simulink model "w2Problem2"  (R2020b)
settings: Solver=ode23  StartTime=0.0  StopTime=10.0  RelTol=1e-3
PostLoadFcn:
  | open_Building_a_Clutch_Lock_Up_Model
undefined symbols (not defined in the file): be, bv, Ie, Iv, muk, mus, R
CloseFcn:
  | close open_Building_a_Clutch_Lock_Up_Model
settings Model: DataDictionary=w2p2_data.sldd  Creator=k.Raviteja  LastModifiedBy=k.Raviteja
settings SolverCC: ZeroCrossAlgorithm=Adaptive
settings DebuggingCC: MaskedZcDiagnostic=none  IgnoredZcDiagnostic=none

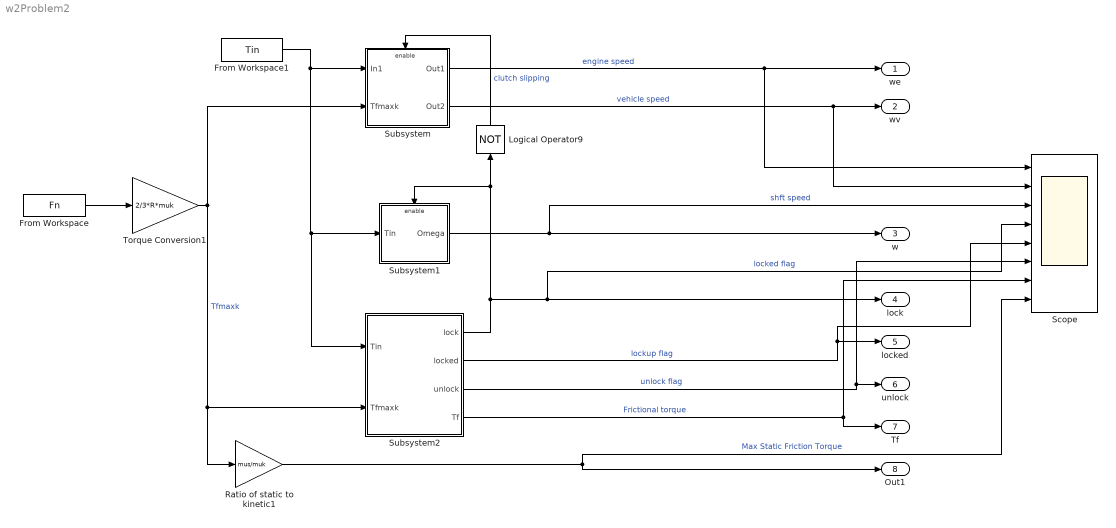
== system w2Problem2 ==
  From Workspace : FromWorkspace  VariableName=Fn  ZeroCross=off
  From Workspace1 : FromWorkspace  VariableName=Tin  ZeroCross=off
  Logical Operator9 : Logic  Operator=NOT  Inputs=1  IconShape=distinctive  OutDataTypeStr=boolean
  Ratio of static to kinetic1 : Gain  Gain=mus/muk  SaturateOnIntegerOverflow=on  OutDataTypeStr=Inherit: Same as input  ParamDataTypeStr=Inherit: Same as input
  Scope : Scope  NumInputPorts=8
  Subsystem : Subsystem
  Subsystem1 : Subsystem
  Subsystem2 : Subsystem
  Torque Conversion1 : Gain  Gain=2/3*R*muk  SaturateOnIntegerOverflow=on  OutDataTypeStr=Inherit: Same as input  ParamDataTypeStr=Inherit: Same as input
  we : Outport  InitialOutput=0  VectorParamsAs1DForOutWhenUnconnected=off
  wv : Outport  Port=2  InitialOutput=0  VectorParamsAs1DForOutWhenUnconnected=off
  w : Outport  Port=3
  lock : Outport  Port=4
  locked : Outport  Port=5
  unlock : Outport  Port=6
  Tf : Outport  Port=7
  Out1 : Outport  Port=8
  wires:
  From Workspace/1 -> Torque Conversion1/1
  Torque Conversion1/1 -> Ratio of static to kinetic1/1, Subsystem2/2(Tfmaxk), Subsystem/2(Tfmaxk)  "Tfmaxk"
  Ratio of static to kinetic1/1 -> Out1/1, Scope/8  "Max Static Friction Torque"
  Subsystem/1(Out1) -> Scope/1, we/1  "engine speed"
  Subsystem/2(Out2) -> Scope/2, wv/1  "vehicle speed"
  Logical Operator9/1 -> Subsystem/Enable  "clutch slipping"
  Subsystem1/1(Omega) -> Scope/3, w/1  "shft speed"
  Subsystem2/1(lock) -> Scope/4, lock/1, Subsystem1/Enable, Logical Operator9/1  "locked flag"
  From Workspace1/1 -> Subsystem2/1(Tin), Subsystem1/1(Tin), Subsystem/1(In1)
  Subsystem2/2(locked) -> Scope/5, locked/1  "lockup flag"
  Subsystem2/3(unlock) -> Scope/6, unlock/1  "unlock flag"
  Subsystem2/4(Tf) -> Tf/1, Scope/7  "Frictional torque"

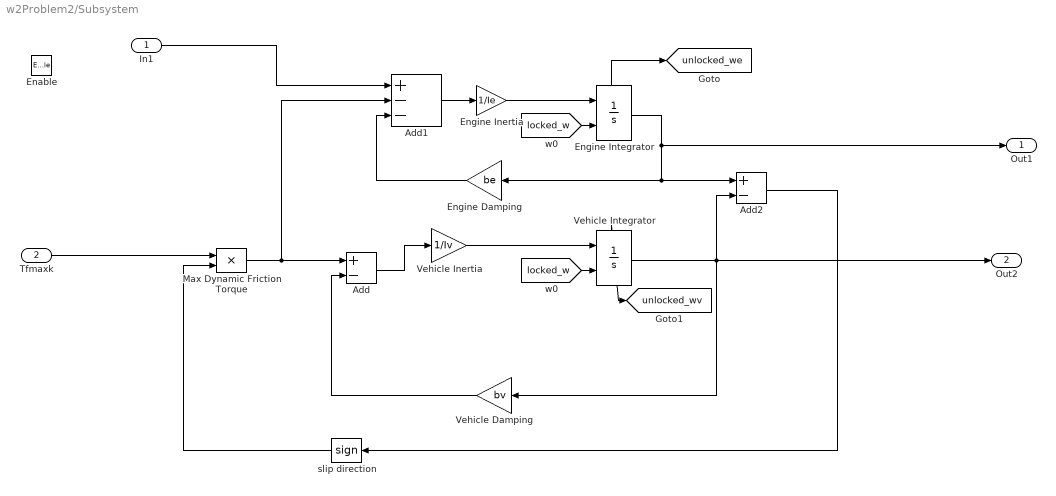
== system w2Problem2/Subsystem ==
  In1 : Inport
  Tfmaxk : Inport  Port=2
  Enable : EnablePort  StatesWhenEnabling=reset
  Add : Sum  Inputs=+-
  Add1 : Sum  Inputs=+--
  Add2 : Sum  Inputs=+-
  Engine Damping : Gain  Gain=be  SaturateOnIntegerOverflow=on  OutDataTypeStr=Inherit: Same as input  ParamDataTypeStr=Inherit: Same as input
  Engine Inertia : Gain  Gain=1/Ie  SaturateOnIntegerOverflow=on  OutDataTypeStr=Inherit: Same as input  ParamDataTypeStr=Inherit: Same as input
  Engine Integrator : Integrator  InitialConditionSource=external  ShowStatePort=on
  Max Dynamic Friction Torque : Product  InputSameDT=on  RndMeth=Zero  SaturateOnIntegerOverflow=on  OutDataTypeStr=Inherit: Same as first input
  Vehicle Damping : Gain  Gain=bv  SaturateOnIntegerOverflow=on  OutDataTypeStr=Inherit: Same as input  ParamDataTypeStr=Inherit: Same as input
  Vehicle Inertia : Gain  Gain=1/Iv  SaturateOnIntegerOverflow=on  OutDataTypeStr=Inherit: Same as input  ParamDataTypeStr=Inherit: Same as input
  Vehicle Integrator : Integrator  InitialConditionSource=external  ShowStatePort=on
  slip direction : Signum
  Out1 : Outport
  Out2 : Outport  Port=2
  tag scope: unlocked_we=global, unlocked_wv=global
  wires:
  [locked_w] -> Vehicle Integrator/2
  Engine Integrator/1 -> Out1/1, Engine Damping/1, Add2/1
  Vehicle Integrator/State -> [unlocked_wv]
  Engine Damping/1 -> Add1/3
  Add2/1 -> slip direction/1
  Max Dynamic Friction Torque/1 -> Add1/2, Add/1
  Engine Inertia/1 -> Engine Integrator/1
  [locked_w] -> Engine Integrator/2
  Vehicle Inertia/1 -> Vehicle Integrator/1
  Engine Integrator/State -> [unlocked_we]
  slip direction/1 -> Max Dynamic Friction Torque/2
  Vehicle Integrator/1 -> Out2/1, Add2/2, Vehicle Damping/1
  Add1/1 -> Engine Inertia/1
  Vehicle Damping/1 -> Add/2
  Add/1 -> Vehicle Inertia/1
  In1/1 -> Add1/1
  Tfmaxk/1 -> Max Dynamic Friction Torque/1

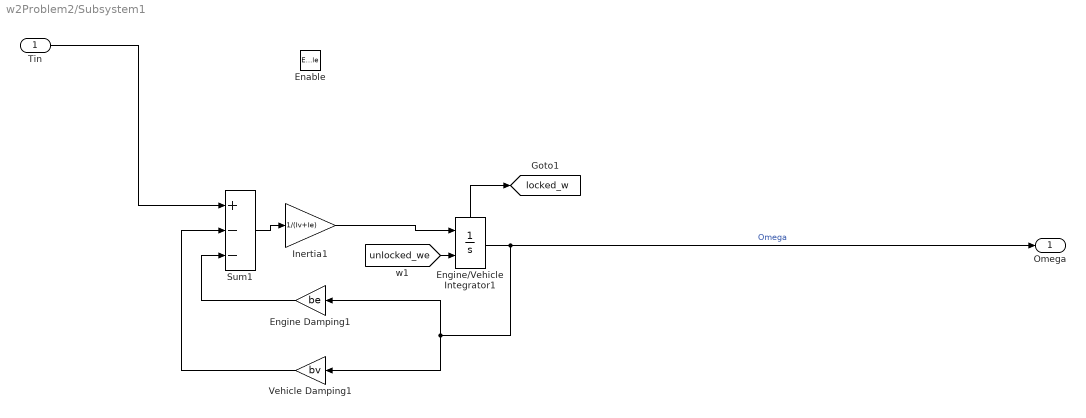
== system w2Problem2/Subsystem1 ==
  Tin : Inport
  Enable : EnablePort  StatesWhenEnabling=reset
  Engine Damping1 : Gain  Gain=be  SaturateOnIntegerOverflow=on  OutDataTypeStr=Inherit: Same as input  ParamDataTypeStr=Inherit: Same as input
  Engine/Vehicle Integrator1 : Integrator  InitialConditionSource=external  ShowStatePort=on
  Inertia1 : Gain  Gain=1/(Iv+Ie)  SaturateOnIntegerOverflow=on  OutDataTypeStr=Inherit: Same as input  ParamDataTypeStr=Inherit: Same as input
  Sum1 : Sum  Inputs=+--  InputSameDT=on  SaturateOnIntegerOverflow=on  OutDataTypeStr=Inherit: Same as first input
  Vehicle Damping1 : Gain  Gain=bv  SaturateOnIntegerOverflow=on  OutDataTypeStr=Inherit: Same as input  ParamDataTypeStr=Inherit: Same as input
  Omega : Outport
  tag scope: locked_w=global
  wires:
  Engine/Vehicle Integrator1/1 -> Omega/1, Engine Damping1/1, Vehicle Damping1/1  "Omega"
  [unlocked_we] -> Engine/Vehicle Integrator1/2
  Sum1/1 -> Inertia1/1
  Engine/Vehicle Integrator1/State -> [locked_w]
  Vehicle Damping1/1 -> Sum1/2
  Engine Damping1/1 -> Sum1/3
  Inertia1/1 -> Engine/Vehicle Integrator1/1
  Tin/1 -> Sum1/1

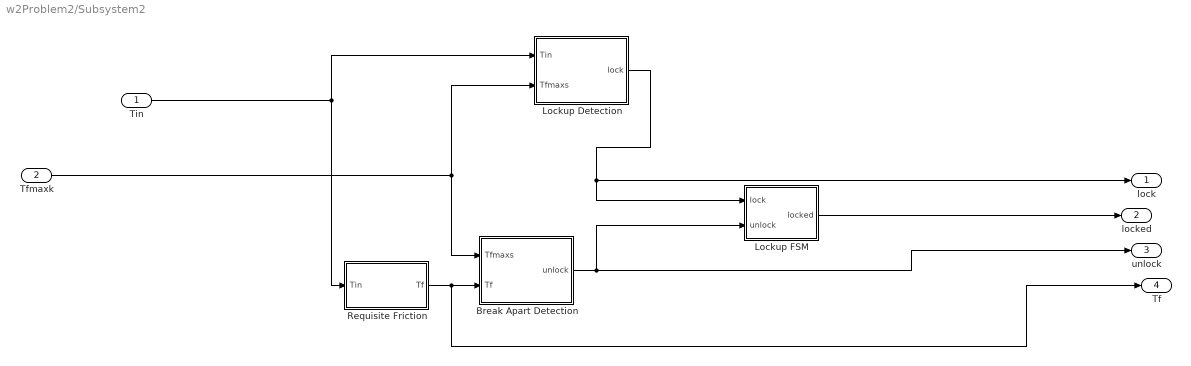
== system w2Problem2/Subsystem2 ==
  Tin : Inport
  Tfmaxk : Inport  Port=2
  Break Apart Detection : Subsystem
  Lockup Detection : Subsystem
  Lockup FSM : Subsystem
  Requisite Friction : Subsystem
  lock : Outport
  locked : Outport  Port=2
  unlock : Outport  Port=3
  Tf : Outport  Port=4
  wires:
  Break Apart Detection/1(unlock) -> unlock/1, Lockup FSM/2(unlock)
  Lockup Detection/1(lock) -> lock/1, Lockup FSM/1(lock)
  Tfmaxk/1 -> Break Apart Detection/1(Tfmaxs), Lockup Detection/2(Tfmaxs)
  Tin/1 -> Requisite Friction/1(Tin), Lockup Detection/1(Tin)
  Requisite Friction/1(Tf) -> Tf/1, Break Apart Detection/2(Tf)
  Lockup FSM/1(locked) -> locked/1

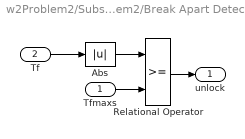
== system w2Problem2/Subsystem2/Break Apart Detection ==
  Tfmaxs : Inport
  Tf : Inport  Port=2
  Abs : Abs  SaturateOnIntegerOverflow=on
  Relational Operator : RelationalOperator  OutDataTypeStr=boolean  RndMeth=Nearest  InputSameDT=on
  unlock : Outport  InitialOutput=0  VectorParamsAs1DForOutWhenUnconnected=off
  wires:
  Tf/1 -> Abs/1
  Relational Operator/1 -> unlock/1
  Abs/1 -> Relational Operator/1
  Tfmaxs/1 -> Relational Operator/2

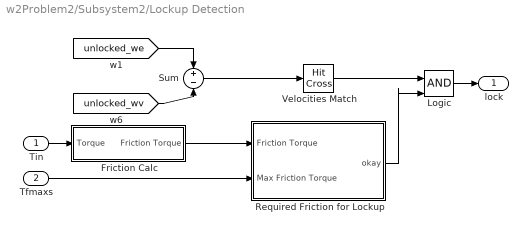
== system w2Problem2/Subsystem2/Lockup Detection ==
  Tin : Inport
  Tfmaxs : Inport  Port=2
  Friction Calc : Subsystem
  Logic : Logic  IconShape=distinctive  OutDataTypeStr=boolean
  Required Friction for Lockup : Subsystem
  Sum : Sum  Inputs=+-  InputSameDT=on  SaturateOnIntegerOverflow=on  OutDataTypeStr=Inherit: Same as first input
  Velocities Match : HitCross
  lock : Outport  InitialOutput=0  VectorParamsAs1DForOutWhenUnconnected=off
  wires:
  Friction Calc/1(Friction Torque) -> Required Friction for Lockup/1(Friction Torque)
  Tfmaxs/1 -> Required Friction for Lockup/2(Max Friction Torque)
  Velocities Match/1 -> Logic/1
  Logic/1 -> lock/1
  Required Friction for Lockup/1(okay) -> Logic/2
  [unlocked_we] -> Sum/1
  [unlocked_wv] -> Sum/2
  Sum/1 -> Velocities Match/1
  Tin/1 -> Friction Calc/1(Torque)

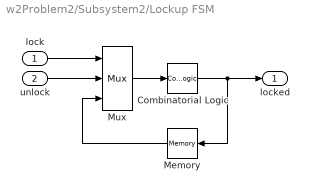
== system w2Problem2/Subsystem2/Lockup FSM ==
  lock : Inport
  unlock : Inport  Port=2
  Combinatorial Logic : CombinatorialLogic  TruthTable=[0;1;0;0;1;1;1;0]
  Memory : Memory
  Mux : Mux  Inputs=3
  locked : Outport  InitialOutput=0  VectorParamsAs1DForOutWhenUnconnected=off
  wires:
  Memory/1 -> Mux/3
  Combinatorial Logic/1 -> locked/1, Memory/1
  unlock/1 -> Mux/2
  lock/1 -> Mux/1
  Mux/1 -> Combinatorial Logic/1

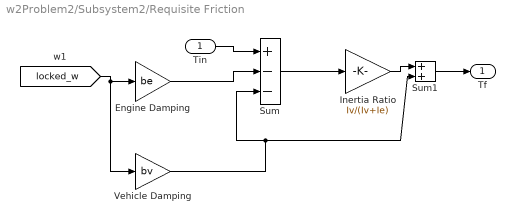
== system w2Problem2/Subsystem2/Requisite Friction ==
  Tin : Inport
  Engine Damping : Gain  Gain=be  SaturateOnIntegerOverflow=on  OutDataTypeStr=Inherit: Same as input  ParamDataTypeStr=Inherit: Same as input
  Inertia Ratio : Gain  Gain=Iv/(Iv+Ie)  SaturateOnIntegerOverflow=on  OutDataTypeStr=Inherit: Same as input  ParamDataTypeStr=Inherit: Same as input
  Sum : Sum  Inputs=+--  InputSameDT=on  SaturateOnIntegerOverflow=on  OutDataTypeStr=Inherit: Same as first input
  Sum1 : Sum  InputSameDT=on  SaturateOnIntegerOverflow=on  OutDataTypeStr=Inherit: Same as first input
  Vehicle Damping : Gain  Gain=bv  SaturateOnIntegerOverflow=on  OutDataTypeStr=Inherit: Same as input  ParamDataTypeStr=Inherit: Same as input
  Tf : Outport  InitialOutput=0  VectorParamsAs1DForOutWhenUnconnected=off
  wires:
  [locked_w] -> Vehicle Damping/1, Engine Damping/1
  Engine Damping/1 -> Sum/2
  Vehicle Damping/1 -> Sum/3, Sum1/2
  Sum/1 -> Inertia Ratio/1
  Tin/1 -> Sum/1
  Inertia Ratio/1 -> Sum1/1
  Sum1/1 -> Tf/1

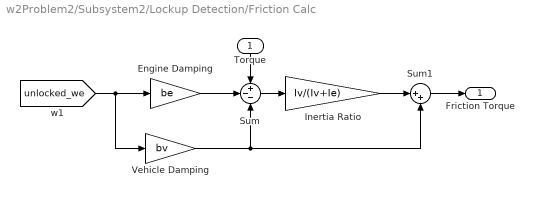
== system w2Problem2/Subsystem2/Lockup Detection/Friction Calc ==
  Torque : Inport
  Engine Damping : Gain  Gain=be  SaturateOnIntegerOverflow=on  OutDataTypeStr=Inherit: Same as input  ParamDataTypeStr=Inherit: Same as input
  Inertia Ratio : Gain  Gain=Iv/(Iv+Ie)  SaturateOnIntegerOverflow=on  OutDataTypeStr=Inherit: Same as input  ParamDataTypeStr=Inherit: Same as input
  Sum : Sum  Inputs=+--  InputSameDT=on  SaturateOnIntegerOverflow=on  OutDataTypeStr=Inherit: Same as first input
  Sum1 : Sum  Inputs=|++  InputSameDT=on  SaturateOnIntegerOverflow=on  OutDataTypeStr=Inherit: Same as first input
  Vehicle Damping : Gain  Gain=bv  SaturateOnIntegerOverflow=on  OutDataTypeStr=Inherit: Same as input  ParamDataTypeStr=Inherit: Same as input
  Friction Torque : Outport  InitialOutput=0  VectorParamsAs1DForOutWhenUnconnected=off
  wires:
  [unlocked_we] -> Engine Damping/1, Vehicle Damping/1
  Vehicle Damping/1 -> Sum1/2, Sum/3
  Engine Damping/1 -> Sum/2
  Sum/1 -> Inertia Ratio/1
  Torque/1 -> Sum/1
  Inertia Ratio/1 -> Sum1/1
  Sum1/1 -> Friction Torque/1

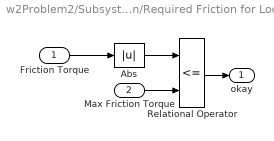
== system w2Problem2/Subsystem2/Lockup Detection/Required Friction for Lockup ==
  Friction Torque : Inport
  Max Friction Torque : Inport  Port=2
  Abs : Abs  SaturateOnIntegerOverflow=on
  Relational Operator : RelationalOperator  Operator=<=  OutDataTypeStr=boolean  RndMeth=Nearest  InputSameDT=on
  okay : Outport  InitialOutput=0  VectorParamsAs1DForOutWhenUnconnected=off
  wires:
  Friction Torque/1 -> Abs/1
  Relational Operator/1 -> okay/1
  Abs/1 -> Relational Operator/1
  Max Friction Torque/1 -> Relational Operator/2
